simulink model "Scenario_13_CoDeSys"  (R2012b)
settings: Solver=ode3  StartTime=0.0  StopTime=inf  FixedStep=Sample_Time_Model  RelTol=1e-3
PreLoadFcn:
  | Variablen_Scenario13
InitFcn:
  | BT = randperm(9);
values from neighbouring files (symbols this model uses):
  Band_Geschwindigkeit = 1.47    [Variablen_Scenario13.m]
  Band_Sensor_Hell_2_Z = -6.5    [Variablen_Scenario13.m]
  Band_Sensor_Hell_3_Z = -10.36    [Variablen_Scenario13.m]
  Band_Sensor_Hell_4_Z = -14.64    [Variablen_Scenario13.m]
  Band_Sensor_Tolerance_Z = 0.2    [Variablen_Scenario13.m]
  Bauteil_Fallgeschwindigkeit = 0.4    [Variablen_Scenario13.m]
  Bauteil_Farbe_Metall = [0.8 0.8 0.8]    [Variablen_Scenario13.m]
  Bauteil_Farbe_Schwarz = [0.2 0.2 0.2]    [Variablen_Scenario13.m]
  Bauteil_Farbe_Weiss = [1 1 0.2]    [Variablen_Scenario13.m]
  Kran_Dauer_90_Grad = 5    [Variablen_Scenario13.m]
  Kran_Drehwinkel_90_Grad = 8050    [Variablen_Scenario13.m]
  Kran_Sensor_Position_Delta = 0.07    [Variablen_Scenario13.m]
  Sample_Time_Model = 0.05    [Variablen_Scenario13.m]
  Sample_Time_Simulation = 0.1    [Variablen_Scenario13.m]
  Sensor_Band_Metall_1 = -6.5    [Variablen_Scenario13.m]
  Sensor_Band_Metall_2 = -10.36    [Variablen_Scenario13.m]
libraries: simulink x557, vrlib x13, opclib x7, rtwinlib x1
(part 6 of 10)

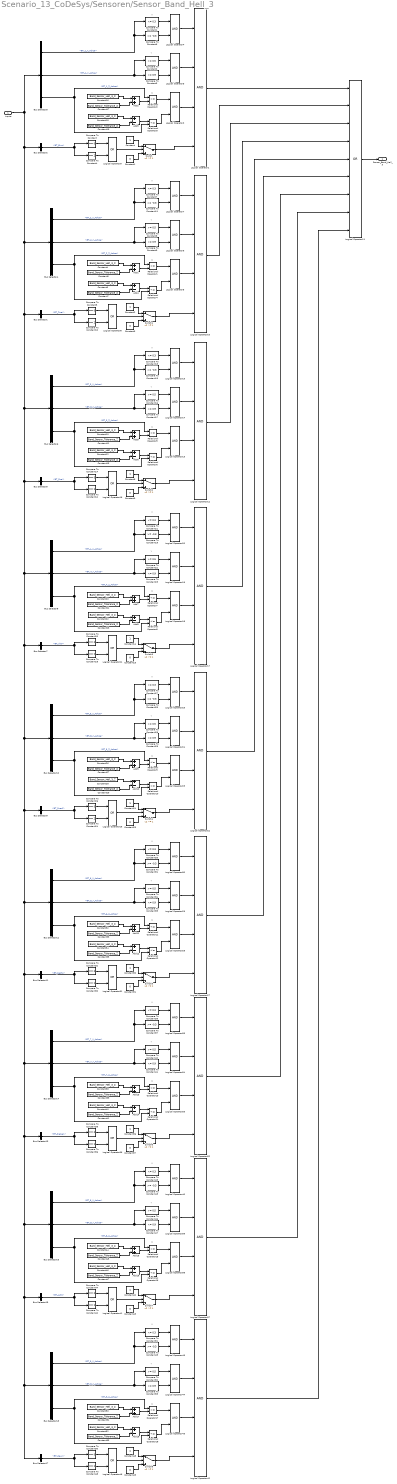
== system Scenario_13_CoDeSys/Sensoren/Sensor_Band_Hell_3 ==
  note: Y
  note: X
  note: Z
  note: Y
  note: X
  note: Z
  note: Y
  note: X
  note: Z
  note: Y
  note: X
  note: Z
  note: Y
  note: X
  note: Z
  note: Y
  note: X
  note: Z
  note: Y
  note: X
  note: Z
  note: Y
  note: X
  note: Z
  note: Y
  note: X
  note: Z
  Inputs : Inport
  Add{1..2,5,7,9,11,13,15,17} (9 alike) : Sum
  Add{3..4,6,8,10,12,14,16,18} (9 alike) : Sum  Inputs=+-
  Bus Selector1 : BusSelector  OutputSignals=Eingaenge.Bauteile.BT_Zwei
  Bus Selector10 : BusSelector  OutputSignals=Bauteil.Stempelanlage_BT.Bauteil_5.BT_5_X_Achse,Bauteil.Stempelanlage_BT.Bauteil_5.BT_5_Y_Achse,Bauteil.Stempelanlage_BT.Bauteil_5.BT_5_Z_Achse
  Bus Selector11 : BusSelector  OutputSignals=Eingaenge.Bauteile.BT_Sechs
  Bus Selector12 : BusSelector  OutputSignals=Bauteil.Stempelanlage_BT.Bauteil_6.BT_6_X_Achse,Bauteil.Stempelanlage_BT.Bauteil_6.BT_6_Y_Achse,Bauteil.Stempelanlage_BT.Bauteil_6.BT_6_Z_Achse
  Bus Selector13 : BusSelector  OutputSignals=Eingaenge.Bauteile.BT_Sieben
  Bus Selector14 : BusSelector  OutputSignals=Bauteil.Stempelanlage_BT.Bauteil_7.BT_7_X_Achse,Bauteil.Stempelanlage_BT.Bauteil_7.BT_7_Y_Achse,Bauteil.Stempelanlage_BT.Bauteil_7.BT_7_Z_Achse
  Bus Selector15 : BusSelector  OutputSignals=Eingaenge.Bauteile.BT_Acht
  Bus Selector16 : BusSelector  OutputSignals=Bauteil.Stempelanlage_BT.Bauteil_8.BT_8_X_Achse,Bauteil.Stempelanlage_BT.Bauteil_8.BT_8_Y_Achse,Bauteil.Stempelanlage_BT.Bauteil_8.BT_8_Z_Achse
  Bus Selector17 : BusSelector  OutputSignals=Eingaenge.Bauteile.BT_Neun
  Bus Selector18 : BusSelector  OutputSignals=Bauteil.Stempelanlage_BT.Bauteil_9.BT_9_X_Achse,Bauteil.Stempelanlage_BT.Bauteil_9.BT_9_Y_Achse,Bauteil.Stempelanlage_BT.Bauteil_9.BT_9_Z_Achse
  Bus Selector2 : BusSelector  OutputSignals=Eingaenge.Bauteile.BT_Eins
  Bus Selector3 : BusSelector  OutputSignals=Bauteil.Stempelanlage_BT.Bauteil_1.BT_1_X_Achse,Bauteil.Stempelanlage_BT.Bauteil_1.BT_1_Y_Achse,Bauteil.Stempelanlage_BT.Bauteil_1.BT_1_Z_Achse
  Bus Selector4 : BusSelector  OutputSignals=Bauteil.Stempelanlage_BT.Bauteil_2.BT_2_X_Achse,Bauteil.Stempelanlage_BT.Bauteil_2.BT_2_Y_Achse,Bauteil.Stempelanlage_BT.Bauteil_2.BT_2_Z_Achse
  Bus Selector5 : BusSelector  OutputSignals=Eingaenge.Bauteile.BT_Drei
  Bus Selector6 : BusSelector  OutputSignals=Bauteil.Stempelanlage_BT.Bauteil_3.BT_3_X_Achse,Bauteil.Stempelanlage_BT.Bauteil_3.BT_3_Y_Achse,Bauteil.Stempelanlage_BT.Bauteil_3.BT_3_Z_Achse
  Bus Selector7 : BusSelector  OutputSignals=Eingaenge.Bauteile.BT_Vier
  Bus Selector8 : BusSelector  OutputSignals=Bauteil.Stempelanlage_BT.Bauteil_4.BT_4_X_Achse,Bauteil.Stempelanlage_BT.Bauteil_4.BT_4_Y_Achse,Bauteil.Stempelanlage_BT.Bauteil_4.BT_4_Z_Achse
  Bus Selector9 : BusSelector  OutputSignals=Eingaenge.Bauteile.BT_Fuenf
  Compare To Constant{,5,14,20,26,32,38,44,50} (9 alike) : simulink/Logic and Bit Operations/Compare To Constant  relop===  const=0  OutDataTypeStr=boolean
  Compare To Constant{1,7,15,21,27,33,39,45,51} (9 alike) : simulink/Logic and Bit Operations/Compare To Constant  relop=<=  const=0.3  OutDataTypeStr=boolean
  Compare To Constant{4,10,12,18,24,30,36,42,48} (9 alike) : simulink/Logic and Bit Operations/Compare To Constant  relop===  const=2  OutDataTypeStr=boolean
  Compare To Constant{6,11,13,19,25,31,37,43,49} (9 alike) : simulink/Logic and Bit Operations/Compare To Constant  relop=>=  const=-0.3  OutDataTypeStr=boolean
  Compare To Constant{2,8,16,22,28,34,40,46,52} (9 alike) : simulink/Logic and Bit Operations/Compare To Constant  relop=>=  const=0.5  OutDataTypeStr=boolean
  Compare To Constant{3,9,17,23,29,35,41,47,53} (9 alike) : simulink/Logic and Bit Operations/Compare To Constant  relop=<=  const=0.9  OutDataTypeStr=boolean
  Constant{,2,8,14,24,30,36,42,48} (9 alike) : Constant
  Constant{1,3,9,15,25,31,37,43,49} (9 alike) : Constant  Value=0
  Constant{4,6,10,12,16,18,20,22,26,28,32,34,38,40,44,46,50,52} (18 alike) : Constant  Value=Band_Sensor_Hell_3_Z
  Constant{5,7,11,13,17,19,21,23,27,29,33,35,39,41,45,47,51,53} (18 alike) : Constant  Value=Band_Sensor_Tolerance_Z
  Logical Operator{1,10,12,17,22,27,32,37,42} (9 alike) : Logic  Inputs=4  AllPortsSameDT=off  OutDataTypeStr=boolean
  Logical Operator11 : Logic  Operator=OR  Inputs=9  AllPortsSameDT=off  OutDataTypeStr=boolean
  Logical Operator{2..7,13..15,18..20,23..25,28..30,33..35,38..40,43..45} (27 alike) : Logic  AllPortsSameDT=off  OutDataTypeStr=boolean
  Logical Operator{8..9,16,21,26,31,36,41,46} (9 alike) : Logic  Operator=OR  AllPortsSameDT=off  OutDataTypeStr=boolean
  Relational Operator{1..18} (18 alike) : RelationalOperator  Operator=<=  OutDataTypeStr=boolean
  Switch{,1..8} (9 alike) : Switch  Threshold=1
  Sensor_Band_Hell_3 : Outport
  wires:
  Bus Selector3/2 -> Compare To Constant2/1, Compare To Constant3/1  "<BT_1_Y_Achse>"
  Compare To Constant2/1 -> Logical Operator3/1
  Compare To Constant3/1 -> Logical Operator3/2
  Logical Operator3/1 -> Logical Operator1/2
  Logical Operator2/1 -> Logical Operator1/3
  Bus Selector3/1 -> Compare To Constant1/1, Compare To Constant6/1  "<BT_1_X_Achse>"
  Compare To Constant1/1 -> Logical Operator4/1
  Compare To Constant6/1 -> Logical Operator4/2
  Logical Operator4/1 -> Logical Operator1/1
  Bus Selector2/1 -> Compare To Constant/1, Compare To Constant4/1  "<BT_Eins>"
  Constant/1 -> Switch/1
  Constant1/1 -> Switch/3
  Relational Operator2/1 -> Logical Operator2/1
  Constant16/1 -> Add2/1
  Constant17/1 -> Add2/2
  Constant18/1 -> Add3/1
  Constant19/1 -> Add3/2
  Add2/1 -> Relational Operator2/2
  Add3/1 -> Relational Operator3/1
  Bus Selector3/3 -> Relational Operator2/1, Relational Operator3/2  "<BT_1_Z_Achse>"
  Relational Operator3/1 -> Logical Operator2/2
  Compare To Constant/1 -> Logical Operator9/1
  Compare To Constant4/1 -> Logical Operator9/2
  Logical Operator9/1 -> Switch/2
  Switch/1 -> Logical Operator1/4
  Compare To Constant8/1 -> Logical Operator6/1
  Compare To Constant9/1 -> Logical Operator6/2
  Logical Operator6/1 -> Logical Operator10/2
  Logical Operator5/1 -> Logical Operator10/3
  Bus Selector4/1 -> Compare To Constant7/1, Compare To Constant11/1  "<BT_2_X_Achse>"
  Compare To Constant7/1 -> Logical Operator7/1
  Compare To Constant11/1 -> Logical Operator7/2
  Logical Operator7/1 -> Logical Operator10/1
  Bus Selector1/1 -> Compare To Constant5/1, Compare To Constant10/1  "<BT_Zwei>"
  Constant2/1 -> Switch1/1
  Constant3/1 -> Switch1/3
  Relational Operator1/1 -> Logical Operator5/1
  Constant4/1 -> Add1/1
  Constant5/1 -> Add1/2
  Constant6/1 -> Add4/1
  Constant7/1 -> Add4/2
  Add1/1 -> Relational Operator1/2
  Add4/1 -> Relational Operator4/1
  Bus Selector4/3 -> Relational Operator1/1, Relational Operator4/2  "<BT_2_Z_Achse>"
  Relational Operator4/1 -> Logical Operator5/2
  Compare To Constant5/1 -> Logical Operator8/1
  Compare To Constant10/1 -> Logical Operator8/2
  Logical Operator8/1 -> Switch1/2
  Switch1/1 -> Logical Operator10/4
  Bus Selector4/2 -> Compare To Constant8/1, Compare To Constant9/1  "<BT_2_Y_Achse>"
  Logical Operator11/1 -> Sensor_Band_Hell_3/1
  Logical Operator1/1 -> Logical Operator11/1
  Logical Operator10/1 -> Logical Operator11/2
  Compare To Constant16/1 -> Logical Operator14/1
  Compare To Constant17/1 -> Logical Operator14/2
  Logical Operator14/1 -> Logical Operator12/2
  Logical Operator13/1 -> Logical Operator12/3
  Bus Selector6/1 -> Compare To Constant15/1, Compare To Constant13/1  "<BT_3_X_Achse>"
  Compare To Constant15/1 -> Logical Operator15/1
  Compare To Constant13/1 -> Logical Operator15/2
  Logical Operator15/1 -> Logical Operator12/1
  Bus Selector5/1 -> Compare To Constant14/1, Compare To Constant12/1  "<BT_Drei>"
  Constant8/1 -> Switch2/1
  Constant9/1 -> Switch2/3
  Relational Operator5/1 -> Logical Operator13/1
  Constant10/1 -> Add5/1
  Constant11/1 -> Add5/2
  Constant12/1 -> Add6/1
  Constant13/1 -> Add6/2
  Add5/1 -> Relational Operator5/2
  Add6/1 -> Relational Operator6/1
  Bus Selector6/3 -> Relational Operator5/1, Relational Operator6/2  "<BT_3_Z_Achse>"
  Relational Operator6/1 -> Logical Operator13/2
  Compare To Constant14/1 -> Logical Operator16/1
  Compare To Constant12/1 -> Logical Operator16/2
  Logical Operator16/1 -> Switch2/2
  Switch2/1 -> Logical Operator12/4
  Bus Selector6/2 -> Compare To Constant16/1, Compare To Constant17/1  "<BT_3_Y_Achse>"
  Compare To Constant22/1 -> Logical Operator19/1
  Compare To Constant23/1 -> Logical Operator19/2
  Logical Operator19/1 -> Logical Operator17/2
  Logical Operator18/1 -> Logical Operator17/3
  Bus Selector8/1 -> Compare To Constant21/1, Compare To Constant19/1  "<BT_4_X_Achse>"
  Compare To Constant21/1 -> Logical Operator20/1
  Compare To Constant19/1 -> Logical Operator20/2
  Logical Operator20/1 -> Logical Operator17/1
  Bus Selector7/1 -> Compare To Constant20/1, Compare To Constant18/1  "<BT_Vier>"
  Constant14/1 -> Switch3/1
  Constant15/1 -> Switch3/3
  Relational Operator7/1 -> Logical Operator18/1
  Constant20/1 -> Add7/1
  Constant21/1 -> Add7/2
  Constant22/1 -> Add8/1
  Constant23/1 -> Add8/2
  Add7/1 -> Relational Operator7/2
  Add8/1 -> Relational Operator8/1
  Bus Selector8/3 -> Relational Operator7/1, Relational Operator8/2  "<BT_4_Z_Achse>"
  Relational Operator8/1 -> Logical Operator18/2
  Compare To Constant20/1 -> Logical Operator21/1
  Compare To Constant18/1 -> Logical Operator21/2
  Logical Operator21/1 -> Switch3/2
  Switch3/1 -> Logical Operator17/4
  Bus Selector8/2 -> Compare To Constant22/1, Compare To Constant23/1  "<BT_4_Y_Achse>"
  Compare To Constant28/1 -> Logical Operator24/1
  Compare To Constant29/1 -> Logical Operator24/2
  Logical Operator24/1 -> Logical Operator22/2
  Logical Operator23/1 -> Logical Operator22/3
  Bus Selector10/1 -> Compare To Constant27/1, Compare To Constant25/1  "<BT_5_X_Achse>"
  Compare To Constant27/1 -> Logical Operator25/1
  Compare To Constant25/1 -> Logical Operator25/2
  Logical Operator25/1 -> Logical Operator22/1
  Bus Selector9/1 -> Compare To Constant26/1, Compare To Constant24/1  "<BT_Fuenf>"
  Constant24/1 -> Switch4/1
  Constant25/1 -> Switch4/3
  Relational Operator9/1 -> Logical Operator23/1
  Constant26/1 -> Add9/1
  Constant27/1 -> Add9/2
  Constant28/1 -> Add10/1
  Constant29/1 -> Add10/2
  Add9/1 -> Relational Operator9/2
  Add10/1 -> Relational Operator10/1
  Bus Selector10/3 -> Relational Operator9/1, Relational Operator10/2  "<BT_5_Z_Achse>"
  Relational Operator10/1 -> Logical Operator23/2
  Compare To Constant26/1 -> Logical Operator26/1
  Compare To Constant24/1 -> Logical Operator26/2
  Logical Operator26/1 -> Switch4/2
  Switch4/1 -> Logical Operator22/4
  Bus Selector10/2 -> Compare To Constant28/1, Compare To Constant29/1  "<BT_5_Y_Achse>"
  Compare To Constant34/1 -> Logical Operator29/1
  Compare To Constant35/1 -> Logical Operator29/2
  Logical Operator29/1 -> Logical Operator27/2
  Logical Operator28/1 -> Logical Operator27/3
  Bus Selector12/1 -> Compare To Constant33/1, Compare To Constant31/1  "<BT_6_X_Achse>"
  Compare To Constant33/1 -> Logical Operator30/1
  Compare To Constant31/1 -> Logical Operator30/2
  Logical Operator30/1 -> Logical Operator27/1
  Bus Selector11/1 -> Compare To Constant32/1, Compare To Constant30/1  "<BT_Sechs>"
  Constant30/1 -> Switch5/1
  Constant31/1 -> Switch5/3
  Relational Operator11/1 -> Logical Operator28/1
  Constant32/1 -> Add11/1
  Constant33/1 -> Add11/2
  Constant34/1 -> Add12/1
  Constant35/1 -> Add12/2
  Add11/1 -> Relational Operator11/2
  Add12/1 -> Relational Operator12/1
  Bus Selector12/3 -> Relational Operator11/1, Relational Operator12/2  "<BT_6_Z_Achse>"
  Relational Operator12/1 -> Logical Operator28/2
  Compare To Constant32/1 -> Logical Operator31/1
  Compare To Constant30/1 -> Logical Operator31/2
  Logical Operator31/1 -> Switch5/2
  Switch5/1 -> Logical Operator27/4
  Bus Selector12/2 -> Compare To Constant34/1, Compare To Constant35/1  "<BT_6_Y_Achse>"
  Logical Operator12/1 -> Logical Operator11/3
  Logical Operator17/1 -> Logical Operator11/4
  Logical Operator22/1 -> Logical Operator11/5
  Logical Operator27/1 -> Logical Operator11/6
  Inputs/1 -> Bus Selector6/1, Bus Selector5/1, Bus Selector8/1, Bus Selector7/1, Bus Selector10/1, Bus Selector9/1, Bus Selector12/1, Bus Selector14/1, Bus Selector16/1, Bus Selector15/1, Bus Selector17/1, Bus Selector18/1, Bus Selector13/1, Bus Selector11/1, Bus Selector1/1, Bus Selector4/1, Bus Selector2/1, Bus Selector3/1
  Compare To Constant40/1 -> Logical Operator34/1
  Compare To Constant41/1 -> Logical Operator34/2
  Logical Operator34/1 -> Logical Operator32/2
  Logical Operator33/1 -> Logical Operator32/3
  Bus Selector14/1 -> Compare To Constant39/1, Compare To Constant37/1  "<BT_7_X_Achse>"
  Compare To Constant39/1 -> Logical Operator35/1
  Compare To Constant37/1 -> Logical Operator35/2
  Logical Operator35/1 -> Logical Operator32/1
  Bus Selector13/1 -> Compare To Constant38/1, Compare To Constant36/1  "<BT_Sieben>"
  Constant36/1 -> Switch6/1
  Constant37/1 -> Switch6/3
  Relational Operator13/1 -> Logical Operator33/1
  Constant38/1 -> Add13/1
  Constant39/1 -> Add13/2
  Constant40/1 -> Add14/1
  Constant41/1 -> Add14/2
  Add13/1 -> Relational Operator13/2
  Add14/1 -> Relational Operator14/1
  Bus Selector14/3 -> Relational Operator13/1, Relational Operator14/2  "<BT_7_Z_Achse>"
  Relational Operator14/1 -> Logical Operator33/2
  Compare To Constant38/1 -> Logical Operator36/1
  Compare To Constant36/1 -> Logical Operator36/2
  Logical Operator36/1 -> Switch6/2
  Switch6/1 -> Logical Operator32/4
  Bus Selector14/2 -> Compare To Constant40/1, Compare To Constant41/1  "<BT_7_Y_Achse>"
  Compare To Constant46/1 -> Logical Operator39/1
  Compare To Constant47/1 -> Logical Operator39/2
  Logical Operator39/1 -> Logical Operator37/2
  Logical Operator38/1 -> Logical Operator37/3
  Bus Selector16/1 -> Compare To Constant45/1, Compare To Constant43/1  "<BT_8_X_Achse>"
  Compare To Constant45/1 -> Logical Operator40/1
  Compare To Constant43/1 -> Logical Operator40/2
  Logical Operator40/1 -> Logical Operator37/1
  Bus Selector15/1 -> Compare To Constant44/1, Compare To Constant42/1  "<BT_Acht>"
  Constant42/1 -> Switch7/1
  Constant43/1 -> Switch7/3
  Relational Operator15/1 -> Logical Operator38/1
  Constant44/1 -> Add15/1
  Constant45/1 -> Add15/2
  Constant46/1 -> Add16/1
  Constant47/1 -> Add16/2
  Add15/1 -> Relational Operator15/2
  Add16/1 -> Relational Operator16/1
  Bus Selector16/3 -> Relational Operator15/1, Relational Operator16/2  "<BT_8_Z_Achse>"
  Relational Operator16/1 -> Logical Operator38/2
  Compare To Constant44/1 -> Logical Operator41/1
  Compare To Constant42/1 -> Logical Operator41/2
  Logical Operator41/1 -> Switch7/2
  Switch7/1 -> Logical Operator37/4
  Bus Selector16/2 -> Compare To Constant46/1, Compare To Constant47/1  "<BT_8_Y_Achse>"
  Compare To Constant52/1 -> Logical Operator44/1
  Compare To Constant53/1 -> Logical Operator44/2
  Logical Operator44/1 -> Logical Operator42/2
  Logical Operator43/1 -> Logical Operator42/3
  Bus Selector18/1 -> Compare To Constant51/1, Compare To Constant49/1  "<BT_9_X_Achse>"
  Compare To Constant51/1 -> Logical Operator45/1
  Compare To Constant49/1 -> Logical Operator45/2
  Logical Operator45/1 -> Logical Operator42/1
  Bus Selector17/1 -> Compare To Constant50/1, Compare To Constant48/1  "<BT_Neun>"
  Constant48/1 -> Switch8/1
  Constant49/1 -> Switch8/3
  Relational Operator17/1 -> Logical Operator43/1
  Constant50/1 -> Add17/1
  Constant51/1 -> Add17/2
  Constant52/1 -> Add18/1
  Constant53/1 -> Add18/2
  Add17/1 -> Relational Operator17/2
  Add18/1 -> Relational Operator18/1
  Bus Selector18/3 -> Relational Operator17/1, Relational Operator18/2  "<BT_9_Z_Achse>"
  Relational Operator18/1 -> Logical Operator43/2
  Compare To Constant50/1 -> Logical Operator46/1
  Compare To Constant48/1 -> Logical Operator46/2
  Logical Operator46/1 -> Switch8/2
  Switch8/1 -> Logical Operator42/4
  Bus Selector18/2 -> Compare To Constant52/1, Compare To Constant53/1  "<BT_9_Y_Achse>"
  Logical Operator32/1 -> Logical Operator11/7
  Logical Operator37/1 -> Logical Operator11/8
  Logical Operator42/1 -> Logical Operator11/9

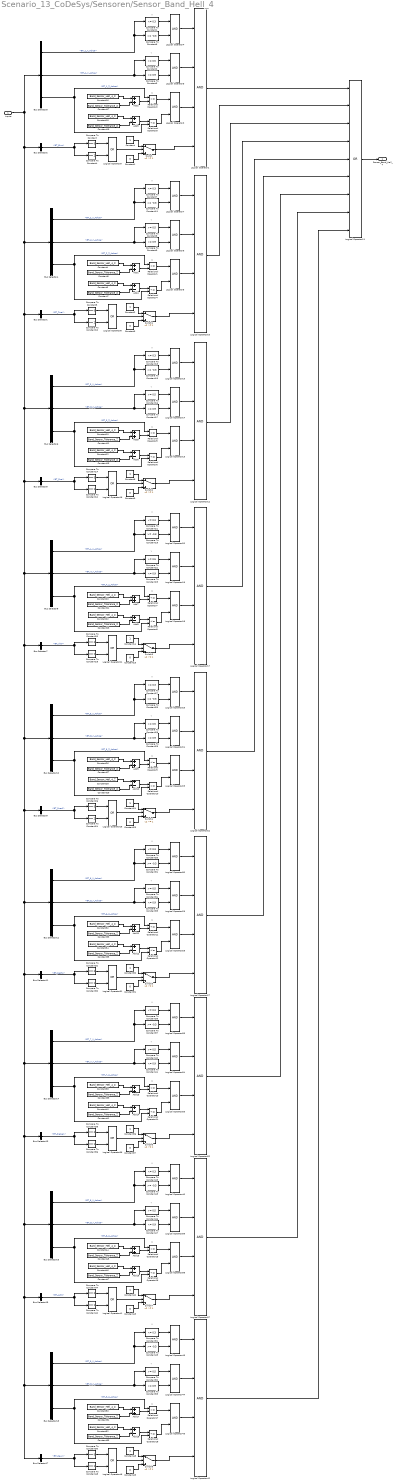
== system Scenario_13_CoDeSys/Sensoren/Sensor_Band_Hell_4 ==
  note: Z
  note: X
  note: Y
  note: Z
  note: X
  note: Y
  note: Z
  note: X
  note: Y
  note: Z
  note: X
  note: Y
  note: Z
  note: X
  note: Y
  note: Z
  note: X
  note: Y
  note: Z
  note: X
  note: Y
  note: Z
  note: X
  note: Y
  note: Z
  note: X
  note: Y
  Inputs : Inport
  Add{1..2,5,7,9,11,13,15,17} (9 alike) : Sum
  Add{3..4,6,8,10,12,14,16,18} (9 alike) : Sum  Inputs=+-
  Bus Selector1 : BusSelector  OutputSignals=Eingaenge.Bauteile.BT_Zwei
  Bus Selector10 : BusSelector  OutputSignals=Bauteil.Stempelanlage_BT.Bauteil_5.BT_5_X_Achse,Bauteil.Stempelanlage_BT.Bauteil_5.BT_5_Y_Achse,Bauteil.Stempelanlage_BT.Bauteil_5.BT_5_Z_Achse
  Bus Selector11 : BusSelector  OutputSignals=Eingaenge.Bauteile.BT_Sechs
  Bus Selector12 : BusSelector  OutputSignals=Bauteil.Stempelanlage_BT.Bauteil_6.BT_6_X_Achse,Bauteil.Stempelanlage_BT.Bauteil_6.BT_6_Y_Achse,Bauteil.Stempelanlage_BT.Bauteil_6.BT_6_Z_Achse
  Bus Selector13 : BusSelector  OutputSignals=Eingaenge.Bauteile.BT_Sieben
  Bus Selector14 : BusSelector  OutputSignals=Bauteil.Stempelanlage_BT.Bauteil_7.BT_7_X_Achse,Bauteil.Stempelanlage_BT.Bauteil_7.BT_7_Y_Achse,Bauteil.Stempelanlage_BT.Bauteil_7.BT_7_Z_Achse
  Bus Selector15 : BusSelector  OutputSignals=Eingaenge.Bauteile.BT_Acht
  Bus Selector16 : BusSelector  OutputSignals=Bauteil.Stempelanlage_BT.Bauteil_8.BT_8_X_Achse,Bauteil.Stempelanlage_BT.Bauteil_8.BT_8_Y_Achse,Bauteil.Stempelanlage_BT.Bauteil_8.BT_8_Z_Achse
  Bus Selector17 : BusSelector  OutputSignals=Eingaenge.Bauteile.BT_Neun
  Bus Selector18 : BusSelector  OutputSignals=Bauteil.Stempelanlage_BT.Bauteil_9.BT_9_X_Achse,Bauteil.Stempelanlage_BT.Bauteil_9.BT_9_Y_Achse,Bauteil.Stempelanlage_BT.Bauteil_9.BT_9_Z_Achse
  Bus Selector2 : BusSelector  OutputSignals=Eingaenge.Bauteile.BT_Eins
  Bus Selector3 : BusSelector  OutputSignals=Bauteil.Stempelanlage_BT.Bauteil_1.BT_1_X_Achse,Bauteil.Stempelanlage_BT.Bauteil_1.BT_1_Y_Achse,Bauteil.Stempelanlage_BT.Bauteil_1.BT_1_Z_Achse
  Bus Selector4 : BusSelector  OutputSignals=Bauteil.Stempelanlage_BT.Bauteil_2.BT_2_X_Achse,Bauteil.Stempelanlage_BT.Bauteil_2.BT_2_Y_Achse,Bauteil.Stempelanlage_BT.Bauteil_2.BT_2_Z_Achse
  Bus Selector5 : BusSelector  OutputSignals=Eingaenge.Bauteile.BT_Drei
  Bus Selector6 : BusSelector  OutputSignals=Bauteil.Stempelanlage_BT.Bauteil_3.BT_3_X_Achse,Bauteil.Stempelanlage_BT.Bauteil_3.BT_3_Y_Achse,Bauteil.Stempelanlage_BT.Bauteil_3.BT_3_Z_Achse
  Bus Selector7 : BusSelector  OutputSignals=Eingaenge.Bauteile.BT_Vier
  Bus Selector8 : BusSelector  OutputSignals=Bauteil.Stempelanlage_BT.Bauteil_4.BT_4_X_Achse,Bauteil.Stempelanlage_BT.Bauteil_4.BT_4_Y_Achse,Bauteil.Stempelanlage_BT.Bauteil_4.BT_4_Z_Achse
  Bus Selector9 : BusSelector  OutputSignals=Eingaenge.Bauteile.BT_Fuenf
  Compare To Constant{,5,14,20,26,32,38,44,50} (9 alike) : simulink/Logic and Bit Operations/Compare To Constant  relop===  const=0  OutDataTypeStr=boolean
  Compare To Constant{1,7,15,21,27,33,39,45,51} (9 alike) : simulink/Logic and Bit Operations/Compare To Constant  relop=<=  const=0.3  OutDataTypeStr=boolean
  Compare To Constant{4,10,12,18,24,30,36,42,48} (9 alike) : simulink/Logic and Bit Operations/Compare To Constant  relop===  const=2  OutDataTypeStr=boolean
  Compare To Constant{6,11,13,19,25,31,37,43,49} (9 alike) : simulink/Logic and Bit Operations/Compare To Constant  relop=>=  const=-0.3  OutDataTypeStr=boolean
  Compare To Constant{2,8,16,22,28,34,40,46,52} (9 alike) : simulink/Logic and Bit Operations/Compare To Constant  relop=>=  const=0.5  OutDataTypeStr=boolean
  Compare To Constant{3,9,17,23,29,35,41,47,53} (9 alike) : simulink/Logic and Bit Operations/Compare To Constant  relop=<=  const=0.9  OutDataTypeStr=boolean
  Constant{,2,8,14,24,30,36,42,48} (9 alike) : Constant
  Constant{1,3,9,15,25,31,37,43,49} (9 alike) : Constant  Value=0
  Constant{4,6,10,12,16,18,20,22,26,28,32,34,38,40,44,46,50,52} (18 alike) : Constant  Value=Band_Sensor_Hell_4_Z
  Constant{5,7,11,13,17,19,21,23,27,29,33,35,39,41,45,47,51,53} (18 alike) : Constant  Value=Band_Sensor_Tolerance_Z
  Logical Operator{1,10,12,17,22,27,32,37,42} (9 alike) : Logic  Inputs=4  AllPortsSameDT=off  OutDataTypeStr=boolean
  Logical Operator11 : Logic  Operator=OR  Inputs=9  AllPortsSameDT=off  OutDataTypeStr=boolean
  Logical Operator{2..7,13..15,18..20,23..25,28..30,33..35,38..40,43..45} (27 alike) : Logic  AllPortsSameDT=off  OutDataTypeStr=boolean
  Logical Operator{8..9,16,21,26,31,36,41,46} (9 alike) : Logic  Operator=OR  AllPortsSameDT=off  OutDataTypeStr=boolean
  Relational Operator{1..18} (18 alike) : RelationalOperator  Operator=<=  OutDataTypeStr=boolean
  Switch{,1..8} (9 alike) : Switch  Threshold=1
  Sensor_Band_Hell_4 : Outport
  wires:
  Logical Operator42/1 -> Logical Operator11/9
  Logical Operator37/1 -> Logical Operator11/8
  Logical Operator32/1 -> Logical Operator11/7
  Bus Selector18/2 -> Compare To Constant53/1, Compare To Constant52/1  "<BT_9_Y_Achse>"
  Switch8/1 -> Logical Operator42/4
  Logical Operator46/1 -> Switch8/2
  Compare To Constant48/1 -> Logical Operator46/2
  Compare To Constant50/1 -> Logical Operator46/1
  Relational Operator18/1 -> Logical Operator43/2
  Bus Selector18/3 -> Relational Operator18/2, Relational Operator17/1  "<BT_9_Z_Achse>"
  Add18/1 -> Relational Operator18/1
  Add17/1 -> Relational Operator17/2
  Constant53/1 -> Add18/2
  Constant52/1 -> Add18/1
  Constant51/1 -> Add17/2
  Constant50/1 -> Add17/1
  Relational Operator17/1 -> Logical Operator43/1
  Constant49/1 -> Switch8/3
  Constant48/1 -> Switch8/1
  Bus Selector17/1 -> Compare To Constant48/1, Compare To Constant50/1  "<BT_Neun>"
  Logical Operator45/1 -> Logical Operator42/1
  Compare To Constant49/1 -> Logical Operator45/2
  Compare To Constant51/1 -> Logical Operator45/1
  Bus Selector18/1 -> Compare To Constant49/1, Compare To Constant51/1  "<BT_9_X_Achse>"
  Logical Operator43/1 -> Logical Operator42/3
  Logical Operator44/1 -> Logical Operator42/2
  Compare To Constant53/1 -> Logical Operator44/2
  Compare To Constant52/1 -> Logical Operator44/1
  Bus Selector16/2 -> Compare To Constant47/1, Compare To Constant46/1  "<BT_8_Y_Achse>"
  Switch7/1 -> Logical Operator37/4
  Logical Operator41/1 -> Switch7/2
  Compare To Constant42/1 -> Logical Operator41/2
  Compare To Constant44/1 -> Logical Operator41/1
  Relational Operator16/1 -> Logical Operator38/2
  Bus Selector16/3 -> Relational Operator16/2, Relational Operator15/1  "<BT_8_Z_Achse>"
  Add16/1 -> Relational Operator16/1
  Add15/1 -> Relational Operator15/2
  Constant47/1 -> Add16/2
  Constant46/1 -> Add16/1
  Constant45/1 -> Add15/2
  Constant44/1 -> Add15/1
  Relational Operator15/1 -> Logical Operator38/1
  Constant43/1 -> Switch7/3
  Constant42/1 -> Switch7/1
  Bus Selector15/1 -> Compare To Constant42/1, Compare To Constant44/1  "<BT_Acht>"
  Logical Operator40/1 -> Logical Operator37/1
  Compare To Constant43/1 -> Logical Operator40/2
  Compare To Constant45/1 -> Logical Operator40/1
  Bus Selector16/1 -> Compare To Constant43/1, Compare To Constant45/1  "<BT_8_X_Achse>"
  Logical Operator38/1 -> Logical Operator37/3
  Logical Operator39/1 -> Logical Operator37/2
  Compare To Constant47/1 -> Logical Operator39/2
  Compare To Constant46/1 -> Logical Operator39/1
  Bus Selector14/2 -> Compare To Constant41/1, Compare To Constant40/1  "<BT_7_Y_Achse>"
  Switch6/1 -> Logical Operator32/4
  Logical Operator36/1 -> Switch6/2
  Compare To Constant36/1 -> Logical Operator36/2
  Compare To Constant38/1 -> Logical Operator36/1
  Relational Operator14/1 -> Logical Operator33/2
  Bus Selector14/3 -> Relational Operator14/2, Relational Operator13/1  "<BT_7_Z_Achse>"
  Add14/1 -> Relational Operator14/1
  Add13/1 -> Relational Operator13/2
  Constant41/1 -> Add14/2
  Constant40/1 -> Add14/1
  Constant39/1 -> Add13/2
  Constant38/1 -> Add13/1
  Relational Operator13/1 -> Logical Operator33/1
  Constant37/1 -> Switch6/3
  Constant36/1 -> Switch6/1
  Bus Selector13/1 -> Compare To Constant36/1, Compare To Constant38/1  "<BT_Sieben>"
  Logical Operator35/1 -> Logical Operator32/1
  Compare To Constant37/1 -> Logical Operator35/2
  Compare To Constant39/1 -> Logical Operator35/1
  Bus Selector14/1 -> Compare To Constant37/1, Compare To Constant39/1  "<BT_7_X_Achse>"
  Logical Operator33/1 -> Logical Operator32/3
  Logical Operator34/1 -> Logical Operator32/2
  Compare To Constant41/1 -> Logical Operator34/2
  Compare To Constant40/1 -> Logical Operator34/1
  Inputs/1 -> Bus Selector3/1, Bus Selector2/1, Bus Selector4/1, Bus Selector1/1, Bus Selector11/1, Bus Selector13/1, Bus Selector18/1, Bus Selector17/1, Bus Selector15/1, Bus Selector16/1, Bus Selector14/1, Bus Selector12/1, Bus Selector9/1, Bus Selector10/1, Bus Selector7/1, Bus Selector8/1, Bus Selector5/1, Bus Selector6/1
  Logical Operator27/1 -> Logical Operator11/6
  Logical Operator22/1 -> Logical Operator11/5
  Logical Operator17/1 -> Logical Operator11/4
  Logical Operator12/1 -> Logical Operator11/3
  Bus Selector12/2 -> Compare To Constant35/1, Compare To Constant34/1  "<BT_6_Y_Achse>"
  Switch5/1 -> Logical Operator27/4
  Logical Operator31/1 -> Switch5/2
  Compare To Constant30/1 -> Logical Operator31/2
  Compare To Constant32/1 -> Logical Operator31/1
  Relational Operator12/1 -> Logical Operator28/2
  Bus Selector12/3 -> Relational Operator12/2, Relational Operator11/1  "<BT_6_Z_Achse>"
  Add12/1 -> Relational Operator12/1
  Add11/1 -> Relational Operator11/2
  Constant35/1 -> Add12/2
  Constant34/1 -> Add12/1
  Constant33/1 -> Add11/2
  Constant32/1 -> Add11/1
  Relational Operator11/1 -> Logical Operator28/1
  Constant31/1 -> Switch5/3
  Constant30/1 -> Switch5/1
  Bus Selector11/1 -> Compare To Constant30/1, Compare To Constant32/1  "<BT_Sechs>"
  Logical Operator30/1 -> Logical Operator27/1
  Compare To Constant31/1 -> Logical Operator30/2
  Compare To Constant33/1 -> Logical Operator30/1
  Bus Selector12/1 -> Compare To Constant31/1, Compare To Constant33/1  "<BT_6_X_Achse>"
  Logical Operator28/1 -> Logical Operator27/3
  Logical Operator29/1 -> Logical Operator27/2
  Compare To Constant35/1 -> Logical Operator29/2
  Compare To Constant34/1 -> Logical Operator29/1
  Bus Selector10/2 -> Compare To Constant29/1, Compare To Constant28/1  "<BT_5_Y_Achse>"
  Switch4/1 -> Logical Operator22/4
  Logical Operator26/1 -> Switch4/2
  Compare To Constant24/1 -> Logical Operator26/2
  Compare To Constant26/1 -> Logical Operator26/1
  Relational Operator10/1 -> Logical Operator23/2
  Bus Selector10/3 -> Relational Operator10/2, Relational Operator9/1  "<BT_5_Z_Achse>"
  Add10/1 -> Relational Operator10/1
  Add9/1 -> Relational Operator9/2
  Constant29/1 -> Add10/2
  Constant28/1 -> Add10/1
  Constant27/1 -> Add9/2
  Constant26/1 -> Add9/1
  Relational Operator9/1 -> Logical Operator23/1
  Constant25/1 -> Switch4/3
  Constant24/1 -> Switch4/1
  Bus Selector9/1 -> Compare To Constant24/1, Compare To Constant26/1  "<BT_Fuenf>"
  Logical Operator25/1 -> Logical Operator22/1
  Compare To Constant25/1 -> Logical Operator25/2
  Compare To Constant27/1 -> Logical Operator25/1
  Bus Selector10/1 -> Compare To Constant25/1, Compare To Constant27/1  "<BT_5_X_Achse>"
  Logical Operator23/1 -> Logical Operator22/3
  Logical Operator24/1 -> Logical Operator22/2
  Compare To Constant29/1 -> Logical Operator24/2
  Compare To Constant28/1 -> Logical Operator24/1
  Bus Selector8/2 -> Compare To Constant23/1, Compare To Constant22/1  "<BT_4_Y_Achse>"
  Switch3/1 -> Logical Operator17/4
  Logical Operator21/1 -> Switch3/2
  Compare To Constant18/1 -> Logical Operator21/2
  Compare To Constant20/1 -> Logical Operator21/1
  Relational Operator8/1 -> Logical Operator18/2
  Bus Selector8/3 -> Relational Operator8/2, Relational Operator7/1  "<BT_4_Z_Achse>"
  Add8/1 -> Relational Operator8/1
  Add7/1 -> Relational Operator7/2
  Constant23/1 -> Add8/2
  Constant22/1 -> Add8/1
  Constant21/1 -> Add7/2
  Constant20/1 -> Add7/1
  Relational Operator7/1 -> Logical Operator18/1
  Constant15/1 -> Switch3/3
  Constant14/1 -> Switch3/1
  Bus Selector7/1 -> Compare To Constant18/1, Compare To Constant20/1  "<BT_Vier>"
  Logical Operator20/1 -> Logical Operator17/1
  Compare To Constant19/1 -> Logical Operator20/2
  Compare To Constant21/1 -> Logical Operator20/1
  Bus Selector8/1 -> Compare To Constant19/1, Compare To Constant21/1  "<BT_4_X_Achse>"
  Logical Operator18/1 -> Logical Operator17/3
  Logical Operator19/1 -> Logical Operator17/2
  Compare To Constant23/1 -> Logical Operator19/2
  Compare To Constant22/1 -> Logical Operator19/1
  Bus Selector6/2 -> Compare To Constant17/1, Compare To Constant16/1  "<BT_3_Y_Achse>"
  Switch2/1 -> Logical Operator12/4
  Logical Operator16/1 -> Switch2/2
  Compare To Constant12/1 -> Logical Operator16/2
  Compare To Constant14/1 -> Logical Operator16/1
  Relational Operator6/1 -> Logical Operator13/2
  Bus Selector6/3 -> Relational Operator6/2, Relational Operator5/1  "<BT_3_Z_Achse>"
  Add6/1 -> Relational Operator6/1
  Add5/1 -> Relational Operator5/2
  Constant13/1 -> Add6/2
  Constant12/1 -> Add6/1
  Constant11/1 -> Add5/2
  Constant10/1 -> Add5/1
  Relational Operator5/1 -> Logical Operator13/1
  Constant9/1 -> Switch2/3
  Constant8/1 -> Switch2/1
  Bus Selector5/1 -> Compare To Constant12/1, Compare To Constant14/1  "<BT_Drei>"
  Logical Operator15/1 -> Logical Operator12/1
  Compare To Constant13/1 -> Logical Operator15/2
  Compare To Constant15/1 -> Logical Operator15/1
  Bus Selector6/1 -> Compare To Constant13/1, Compare To Constant15/1  "<BT_3_X_Achse>"
  Logical Operator13/1 -> Logical Operator12/3
  Logical Operator14/1 -> Logical Operator12/2
  Compare To Constant17/1 -> Logical Operator14/2
  Compare To Constant16/1 -> Logical Operator14/1
  Logical Operator10/1 -> Logical Operator11/2
  Logical Operator1/1 -> Logical Operator11/1
  Logical Operator11/1 -> Sensor_Band_Hell_4/1
  Bus Selector4/2 -> Compare To Constant9/1, Compare To Constant8/1  "<BT_2_Y_Achse>"
  Switch1/1 -> Logical Operator10/4
  Logical Operator8/1 -> Switch1/2
  Compare To Constant10/1 -> Logical Operator8/2
  Compare To Constant5/1 -> Logical Operator8/1
  Relational Operator4/1 -> Logical Operator5/2
  Bus Selector4/3 -> Relational Operator4/2, Relational Operator1/1  "<BT_2_Z_Achse>"
  Add4/1 -> Relational Operator4/1
  Add1/1 -> Relational Operator1/2
  Constant7/1 -> Add4/2
  Constant6/1 -> Add4/1
  Constant5/1 -> Add1/2
  Constant4/1 -> Add1/1
  Relational Operator1/1 -> Logical Operator5/1
  Constant3/1 -> Switch1/3
  Constant2/1 -> Switch1/1
  Bus Selector1/1 -> Compare To Constant10/1, Compare To Constant5/1  "<BT_Zwei>"
  Logical Operator7/1 -> Logical Operator10/1
  Compare To Constant11/1 -> Logical Operator7/2
  Compare To Constant7/1 -> Logical Operator7/1
  Bus Selector4/1 -> Compare To Constant11/1, Compare To Constant7/1  "<BT_2_X_Achse>"
  Logical Operator5/1 -> Logical Operator10/3
  Logical Operator6/1 -> Logical Operator10/2
  Compare To Constant9/1 -> Logical Operator6/2
  Compare To Constant8/1 -> Logical Operator6/1
  Switch/1 -> Logical Operator1/4
  Logical Operator9/1 -> Switch/2
  Compare To Constant4/1 -> Logical Operator9/2
  Compare To Constant/1 -> Logical Operator9/1
  Relational Operator3/1 -> Logical Operator2/2
  Bus Selector3/3 -> Relational Operator3/2, Relational Operator2/1  "<BT_1_Z_Achse>"
  Add3/1 -> Relational Operator3/1
  Add2/1 -> Relational Operator2/2
  Constant19/1 -> Add3/2
  Constant18/1 -> Add3/1
  Constant17/1 -> Add2/2
  Constant16/1 -> Add2/1
  Relational Operator2/1 -> Logical Operator2/1
  Constant1/1 -> Switch/3
  Constant/1 -> Switch/1
  Bus Selector2/1 -> Compare To Constant4/1, Compare To Constant/1  "<BT_Eins>"
  Logical Operator4/1 -> Logical Operator1/1
  Compare To Constant6/1 -> Logical Operator4/2
  Compare To Constant1/1 -> Logical Operator4/1
  Bus Selector3/1 -> Compare To Constant6/1, Compare To Constant1/1  "<BT_1_X_Achse>"
  Logical Operator2/1 -> Logical Operator1/3
  Logical Operator3/1 -> Logical Operator1/2
  Compare To Constant3/1 -> Logical Operator3/2
  Compare To Constant2/1 -> Logical Operator3/1
  Bus Selector3/2 -> Compare To Constant3/1, Compare To Constant2/1  "<BT_1_Y_Achse>"

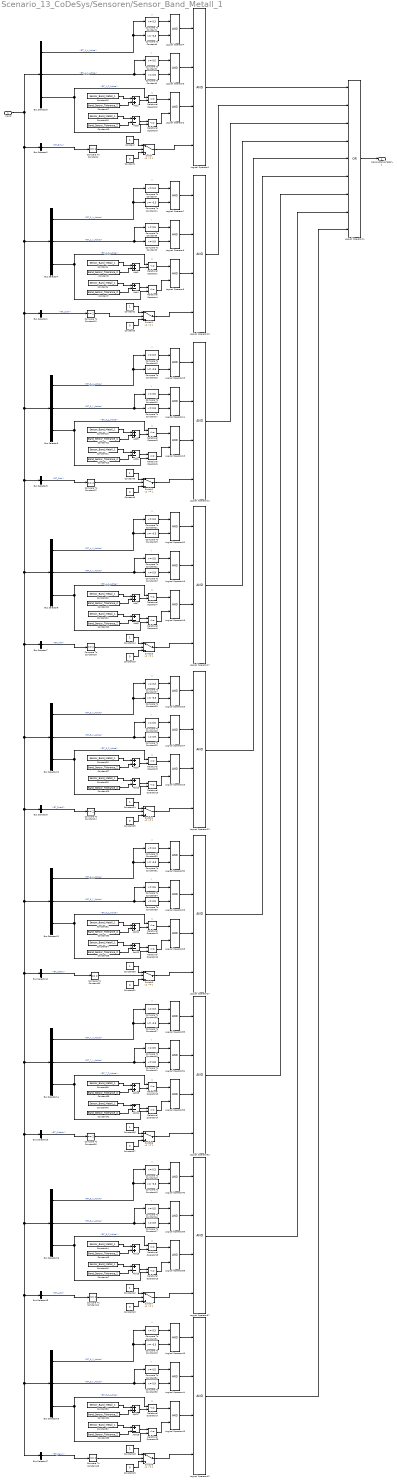
== system Scenario_13_CoDeSys/Sensoren/Sensor_Band_Metall_1 ==
  note: Y
  note: X
  note: Z
  note: Y
  note: X
  note: Z
  note: Y
  note: X
  note: Z
  note: Y
  note: X
  note: Z
  note: Y
  note: X
  note: Z
  note: Y
  note: X
  note: Z
  note: Y
  note: X
  note: Z
  note: Y
  note: X
  note: Z
  note: Y
  note: X
  note: Z
  Inputs : Inport
  Add{1..2,5,7,9,11,13,15,17} (9 alike) : Sum
  Add{3..4,6,8,10,12,14,16,18} (9 alike) : Sum  Inputs=+-
  Bus Selector1 : BusSelector  OutputSignals=Eingaenge.Bauteile.BT_Zwei
  Bus Selector10 : BusSelector  OutputSignals=Bauteil.Stempelanlage_BT.Bauteil_5.BT_5_X_Achse,Bauteil.Stempelanlage_BT.Bauteil_5.BT_5_Y_Achse,Bauteil.Stempelanlage_BT.Bauteil_5.BT_5_Z_Achse
  Bus Selector11 : BusSelector  OutputSignals=Eingaenge.Bauteile.BT_Sechs
  Bus Selector12 : BusSelector  OutputSignals=Bauteil.Stempelanlage_BT.Bauteil_6.BT_6_X_Achse,Bauteil.Stempelanlage_BT.Bauteil_6.BT_6_Y_Achse,Bauteil.Stempelanlage_BT.Bauteil_6.BT_6_Z_Achse
  Bus Selector13 : BusSelector  OutputSignals=Eingaenge.Bauteile.BT_Sieben
  Bus Selector14 : BusSelector  OutputSignals=Bauteil.Stempelanlage_BT.Bauteil_7.BT_7_X_Achse,Bauteil.Stempelanlage_BT.Bauteil_7.BT_7_Y_Achse,Bauteil.Stempelanlage_BT.Bauteil_7.BT_7_Z_Achse
  Bus Selector15 : BusSelector  OutputSignals=Eingaenge.Bauteile.BT_Acht
  Bus Selector16 : BusSelector  OutputSignals=Bauteil.Stempelanlage_BT.Bauteil_8.BT_8_X_Achse,Bauteil.Stempelanlage_BT.Bauteil_8.BT_8_Y_Achse,Bauteil.Stempelanlage_BT.Bauteil_8.BT_8_Z_Achse
  Bus Selector17 : BusSelector  OutputSignals=Eingaenge.Bauteile.BT_Neun
  Bus Selector18 : BusSelector  OutputSignals=Bauteil.Stempelanlage_BT.Bauteil_9.BT_9_X_Achse,Bauteil.Stempelanlage_BT.Bauteil_9.BT_9_Y_Achse,Bauteil.Stempelanlage_BT.Bauteil_9.BT_9_Z_Achse
  Bus Selector2 : BusSelector  OutputSignals=Eingaenge.Bauteile.BT_Eins
  Bus Selector3 : BusSelector  OutputSignals=Bauteil.Stempelanlage_BT.Bauteil_1.BT_1_X_Achse,Bauteil.Stempelanlage_BT.Bauteil_1.BT_1_Y_Achse,Bauteil.Stempelanlage_BT.Bauteil_1.BT_1_Z_Achse
  Bus Selector4 : BusSelector  OutputSignals=Bauteil.Stempelanlage_BT.Bauteil_2.BT_2_X_Achse,Bauteil.Stempelanlage_BT.Bauteil_2.BT_2_Y_Achse,Bauteil.Stempelanlage_BT.Bauteil_2.BT_2_Z_Achse
  Bus Selector5 : BusSelector  OutputSignals=Eingaenge.Bauteile.BT_Drei
  Bus Selector6 : BusSelector  OutputSignals=Bauteil.Stempelanlage_BT.Bauteil_3.BT_3_X_Achse,Bauteil.Stempelanlage_BT.Bauteil_3.BT_3_Y_Achse,Bauteil.Stempelanlage_BT.Bauteil_3.BT_3_Z_Achse
  Bus Selector7 : BusSelector  OutputSignals=Eingaenge.Bauteile.BT_Vier
  Bus Selector8 : BusSelector  OutputSignals=Bauteil.Stempelanlage_BT.Bauteil_4.BT_4_X_Achse,Bauteil.Stempelanlage_BT.Bauteil_4.BT_4_Y_Achse,Bauteil.Stempelanlage_BT.Bauteil_4.BT_4_Z_Achse
  Bus Selector9 : BusSelector  OutputSignals=Eingaenge.Bauteile.BT_Fuenf
  Compare To Constant{1,7,15,21,27,33,39,45,51} (9 alike) : simulink/Logic and Bit Operations/Compare To Constant  relop=<=  const=0.3  OutDataTypeStr=boolean
  Compare To Constant{4,10,12,18,24,30,36,42,48} (9 alike) : simulink/Logic and Bit Operations/Compare To Constant  relop===  const=2  OutDataTypeStr=boolean
  Compare To Constant{6,11,13,19,25,31,37,43,49} (9 alike) : simulink/Logic and Bit Operations/Compare To Constant  relop=>=  const=-0.3  OutDataTypeStr=boolean
  Compare To Constant{2,8,16,22,28,34,40,46,52} (9 alike) : simulink/Logic and Bit Operations/Compare To Constant  relop=>=  const=0.5  OutDataTypeStr=boolean
  Compare To Constant{3,9,17,23,29,35,41,47,53} (9 alike) : simulink/Logic and Bit Operations/Compare To Constant  relop=<=  const=0.9  OutDataTypeStr=boolean
  Constant{,2,8,14,24,30,36,42,48} (9 alike) : Constant
  Constant{1,3,9,15,25,31,37,43,49} (9 alike) : Constant  Value=0
  Constant{4,6,10,12,16,18,20,22,26,28,32,34,38,40,44,46,50,52} (18 alike) : Constant  Value=Sensor_Band_Metall_1
  Constant{5,7,11,13,17,19,21,23,27,29,33,35,39,41,45,47,51,53} (18 alike) : Constant  Value=Band_Sensor_Tolerance_Z
  Logical Operator{1,10,12,17,22,27,32,37,42} (9 alike) : Logic  Inputs=4  AllPortsSameDT=off  OutDataTypeStr=boolean
  Logical Operator11 : Logic  Operator=OR  Inputs=9  AllPortsSameDT=off  OutDataTypeStr=boolean
  Logical Operator{2..7,13..15,18..20,23..25,28..30,33..35,38..40,43..45} (27 alike) : Logic  AllPortsSameDT=off  OutDataTypeStr=boolean
  Relational Operator{1..18} (18 alike) : RelationalOperator  Operator=<=  OutDataTypeStr=boolean
  Switch{,1..8} (9 alike) : Switch  Threshold=1
  Sensor_Band_Metall_1 : Outport
  wires:
  Bus Selector3/2 -> Compare To Constant2/1, Compare To Constant3/1  "<BT_1_Y_Achse>"
  Compare To Constant2/1 -> Logical Operator3/1
  Compare To Constant3/1 -> Logical Operator3/2
  Logical Operator3/1 -> Logical Operator1/2
  Logical Operator2/1 -> Logical Operator1/3
  Bus Selector3/1 -> Compare To Constant1/1, Compare To Constant6/1  "<BT_1_X_Achse>"
  Compare To Constant1/1 -> Logical Operator4/1
  Compare To Constant6/1 -> Logical Operator4/2
  Logical Operator4/1 -> Logical Operator1/1
  Bus Selector2/1 -> Compare To Constant4/1  "<BT_Eins>"
  Constant/1 -> Switch/1
  Constant1/1 -> Switch/3
  Relational Operator2/1 -> Logical Operator2/1
  Constant16/1 -> Add2/1
  Constant17/1 -> Add2/2
  Constant18/1 -> Add3/1
  Constant19/1 -> Add3/2
  Add2/1 -> Relational Operator2/2
  Add3/1 -> Relational Operator3/1
  Bus Selector3/3 -> Relational Operator2/1, Relational Operator3/2  "<BT_1_Z_Achse>"
  Relational Operator3/1 -> Logical Operator2/2
  Compare To Constant4/1 -> Switch/2
  Switch/1 -> Logical Operator1/4
  Compare To Constant8/1 -> Logical Operator6/1
  Compare To Constant9/1 -> Logical Operator6/2
  Logical Operator6/1 -> Logical Operator10/2
  Logical Operator5/1 -> Logical Operator10/3
  Bus Selector4/1 -> Compare To Constant7/1, Compare To Constant11/1  "<BT_2_X_Achse>"
  Compare To Constant7/1 -> Logical Operator7/1
  Compare To Constant11/1 -> Logical Operator7/2
  Logical Operator7/1 -> Logical Operator10/1
  Bus Selector1/1 -> Compare To Constant10/1  "<BT_Zwei>"
  Constant2/1 -> Switch1/1
  Constant3/1 -> Switch1/3
  Relational Operator1/1 -> Logical Operator5/1
  Constant4/1 -> Add1/1
  Constant5/1 -> Add1/2
  Constant6/1 -> Add4/1
  Constant7/1 -> Add4/2
  Add1/1 -> Relational Operator1/2
  Add4/1 -> Relational Operator4/1
  Bus Selector4/3 -> Relational Operator1/1, Relational Operator4/2  "<BT_2_Z_Achse>"
  Relational Operator4/1 -> Logical Operator5/2
  Compare To Constant10/1 -> Switch1/2
  Switch1/1 -> Logical Operator10/4
  Bus Selector4/2 -> Compare To Constant8/1, Compare To Constant9/1  "<BT_2_Y_Achse>"
  Logical Operator11/1 -> Sensor_Band_Metall_1/1
  Logical Operator1/1 -> Logical Operator11/1
  Logical Operator10/1 -> Logical Operator11/2
  Compare To Constant16/1 -> Logical Operator14/1
  Compare To Constant17/1 -> Logical Operator14/2
  Logical Operator14/1 -> Logical Operator12/2
  Logical Operator13/1 -> Logical Operator12/3
  Bus Selector6/1 -> Compare To Constant15/1, Compare To Constant13/1  "<BT_3_X_Achse>"
  Compare To Constant15/1 -> Logical Operator15/1
  Compare To Constant13/1 -> Logical Operator15/2
  Logical Operator15/1 -> Logical Operator12/1
  Bus Selector5/1 -> Compare To Constant12/1  "<BT_Drei>"
  Constant8/1 -> Switch2/1
  Constant9/1 -> Switch2/3
  Relational Operator5/1 -> Logical Operator13/1
  Constant10/1 -> Add5/1
  Constant11/1 -> Add5/2
  Constant12/1 -> Add6/1
  Constant13/1 -> Add6/2
  Add5/1 -> Relational Operator5/2
  Add6/1 -> Relational Operator6/1
  Bus Selector6/3 -> Relational Operator5/1, Relational Operator6/2  "<BT_3_Z_Achse>"
  Relational Operator6/1 -> Logical Operator13/2
  Compare To Constant12/1 -> Switch2/2
  Switch2/1 -> Logical Operator12/4
  Bus Selector6/2 -> Compare To Constant16/1, Compare To Constant17/1  "<BT_3_Y_Achse>"
  Compare To Constant22/1 -> Logical Operator19/1
  Compare To Constant23/1 -> Logical Operator19/2
  Logical Operator19/1 -> Logical Operator17/2
  Logical Operator18/1 -> Logical Operator17/3
  Bus Selector8/1 -> Compare To Constant21/1, Compare To Constant19/1  "<BT_4_X_Achse>"
  Compare To Constant21/1 -> Logical Operator20/1
  Compare To Constant19/1 -> Logical Operator20/2
  Logical Operator20/1 -> Logical Operator17/1
  Bus Selector7/1 -> Compare To Constant18/1  "<BT_Vier>"
  Constant14/1 -> Switch3/1
  Constant15/1 -> Switch3/3
  Relational Operator7/1 -> Logical Operator18/1
  Constant20/1 -> Add7/1
  Constant21/1 -> Add7/2
  Constant22/1 -> Add8/1
  Constant23/1 -> Add8/2
  Add7/1 -> Relational Operator7/2
  Add8/1 -> Relational Operator8/1
  Bus Selector8/3 -> Relational Operator7/1, Relational Operator8/2  "<BT_4_Z_Achse>"
  Relational Operator8/1 -> Logical Operator18/2
  Compare To Constant18/1 -> Switch3/2
  Switch3/1 -> Logical Operator17/4
  Bus Selector8/2 -> Compare To Constant22/1, Compare To Constant23/1  "<BT_4_Y_Achse>"
  Compare To Constant28/1 -> Logical Operator24/1
  Compare To Constant29/1 -> Logical Operator24/2
  Logical Operator24/1 -> Logical Operator22/2
  Logical Operator23/1 -> Logical Operator22/3
  Bus Selector10/1 -> Compare To Constant27/1, Compare To Constant25/1  "<BT_5_X_Achse>"
  Compare To Constant27/1 -> Logical Operator25/1
  Compare To Constant25/1 -> Logical Operator25/2
  Logical Operator25/1 -> Logical Operator22/1
  Bus Selector9/1 -> Compare To Constant24/1  "<BT_Fuenf>"
  Constant24/1 -> Switch4/1
  Constant25/1 -> Switch4/3
  Relational Operator9/1 -> Logical Operator23/1
  Constant26/1 -> Add9/1
  Constant27/1 -> Add9/2
  Constant28/1 -> Add10/1
  Constant29/1 -> Add10/2
  Add9/1 -> Relational Operator9/2
  Add10/1 -> Relational Operator10/1
  Bus Selector10/3 -> Relational Operator9/1, Relational Operator10/2  "<BT_5_Z_Achse>"
  Relational Operator10/1 -> Logical Operator23/2
  Compare To Constant24/1 -> Switch4/2
  Switch4/1 -> Logical Operator22/4
  Bus Selector10/2 -> Compare To Constant28/1, Compare To Constant29/1  "<BT_5_Y_Achse>"
  Compare To Constant34/1 -> Logical Operator29/1
  Compare To Constant35/1 -> Logical Operator29/2
  Logical Operator29/1 -> Logical Operator27/2
  Logical Operator28/1 -> Logical Operator27/3
  Bus Selector12/1 -> Compare To Constant33/1, Compare To Constant31/1  "<BT_6_X_Achse>"
  Compare To Constant33/1 -> Logical Operator30/1
  Compare To Constant31/1 -> Logical Operator30/2
  Logical Operator30/1 -> Logical Operator27/1
  Bus Selector11/1 -> Compare To Constant30/1  "<BT_Sechs>"
  Constant30/1 -> Switch5/1
  Constant31/1 -> Switch5/3
  Relational Operator11/1 -> Logical Operator28/1
  Constant32/1 -> Add11/1
  Constant33/1 -> Add11/2
  Constant34/1 -> Add12/1
  Constant35/1 -> Add12/2
  Add11/1 -> Relational Operator11/2
  Add12/1 -> Relational Operator12/1
  Bus Selector12/3 -> Relational Operator11/1, Relational Operator12/2  "<BT_6_Z_Achse>"
  Relational Operator12/1 -> Logical Operator28/2
  Compare To Constant30/1 -> Switch5/2
  Switch5/1 -> Logical Operator27/4
  Bus Selector12/2 -> Compare To Constant34/1, Compare To Constant35/1  "<BT_6_Y_Achse>"
  Logical Operator12/1 -> Logical Operator11/3
  Logical Operator17/1 -> Logical Operator11/4
  Logical Operator22/1 -> Logical Operator11/5
  Logical Operator27/1 -> Logical Operator11/6
  Inputs/1 -> Bus Selector6/1, Bus Selector5/1, Bus Selector8/1, Bus Selector7/1, Bus Selector10/1, Bus Selector9/1, Bus Selector12/1, Bus Selector14/1, Bus Selector16/1, Bus Selector15/1, Bus Selector17/1, Bus Selector18/1, Bus Selector13/1, Bus Selector11/1, Bus Selector1/1, Bus Selector4/1, Bus Selector2/1, Bus Selector3/1
  Compare To Constant40/1 -> Logical Operator34/1
  Compare To Constant41/1 -> Logical Operator34/2
  Logical Operator34/1 -> Logical Operator32/2
  Logical Operator33/1 -> Logical Operator32/3
  Bus Selector14/1 -> Compare To Constant39/1, Compare To Constant37/1  "<BT_7_X_Achse>"
  Compare To Constant39/1 -> Logical Operator35/1
  Compare To Constant37/1 -> Logical Operator35/2
  Logical Operator35/1 -> Logical Operator32/1
  Bus Selector13/1 -> Compare To Constant36/1  "<BT_Sieben>"
  Constant36/1 -> Switch6/1
  Constant37/1 -> Switch6/3
  Relational Operator13/1 -> Logical Operator33/1
  Constant38/1 -> Add13/1
  Constant39/1 -> Add13/2
  Constant40/1 -> Add14/1
  Constant41/1 -> Add14/2
  Add13/1 -> Relational Operator13/2
  Add14/1 -> Relational Operator14/1
  Bus Selector14/3 -> Relational Operator13/1, Relational Operator14/2  "<BT_7_Z_Achse>"
  Relational Operator14/1 -> Logical Operator33/2
  Compare To Constant36/1 -> Switch6/2
  Switch6/1 -> Logical Operator32/4
  Bus Selector14/2 -> Compare To Constant40/1, Compare To Constant41/1  "<BT_7_Y_Achse>"
  Compare To Constant46/1 -> Logical Operator39/1
  Compare To Constant47/1 -> Logical Operator39/2
  Logical Operator39/1 -> Logical Operator37/2
  Logical Operator38/1 -> Logical Operator37/3
  Bus Selector16/1 -> Compare To Constant45/1, Compare To Constant43/1  "<BT_8_X_Achse>"
  Compare To Constant45/1 -> Logical Operator40/1
  Compare To Constant43/1 -> Logical Operator40/2
  Logical Operator40/1 -> Logical Operator37/1
  Bus Selector15/1 -> Compare To Constant42/1  "<BT_Acht>"
  Constant42/1 -> Switch7/1
  Constant43/1 -> Switch7/3
  Relational Operator15/1 -> Logical Operator38/1
  Constant44/1 -> Add15/1
  Constant45/1 -> Add15/2
  Constant46/1 -> Add16/1
  Constant47/1 -> Add16/2
  Add15/1 -> Relational Operator15/2
  Add16/1 -> Relational Operator16/1
  Bus Selector16/3 -> Relational Operator15/1, Relational Operator16/2  "<BT_8_Z_Achse>"
  Relational Operator16/1 -> Logical Operator38/2
  Compare To Constant42/1 -> Switch7/2
  Switch7/1 -> Logical Operator37/4
  Bus Selector16/2 -> Compare To Constant46/1, Compare To Constant47/1  "<BT_8_Y_Achse>"
  Compare To Constant52/1 -> Logical Operator44/1
  Compare To Constant53/1 -> Logical Operator44/2
  Logical Operator44/1 -> Logical Operator42/2
  Logical Operator43/1 -> Logical Operator42/3
  Bus Selector18/1 -> Compare To Constant51/1, Compare To Constant49/1  "<BT_9_X_Achse>"
  Compare To Constant51/1 -> Logical Operator45/1
  Compare To Constant49/1 -> Logical Operator45/2
  Logical Operator45/1 -> Logical Operator42/1
  Bus Selector17/1 -> Compare To Constant48/1  "<BT_Neun>"
  Constant48/1 -> Switch8/1
  Constant49/1 -> Switch8/3
  Relational Operator17/1 -> Logical Operator43/1
  Constant50/1 -> Add17/1
  Constant51/1 -> Add17/2
  Constant52/1 -> Add18/1
  Constant53/1 -> Add18/2
  Add17/1 -> Relational Operator17/2
  Add18/1 -> Relational Operator18/1
  Bus Selector18/3 -> Relational Operator17/1, Relational Operator18/2  "<BT_9_Z_Achse>"
  Relational Operator18/1 -> Logical Operator43/2
  Compare To Constant48/1 -> Switch8/2
  Switch8/1 -> Logical Operator42/4
  Bus Selector18/2 -> Compare To Constant52/1, Compare To Constant53/1  "<BT_9_Y_Achse>"
  Logical Operator32/1 -> Logical Operator11/7
  Logical Operator37/1 -> Logical Operator11/8
  Logical Operator42/1 -> Logical Operator11/9
